simulink model "bpsk_revised"  (R2024a)
settings: Solver=FixedStepAuto  StartTime=0.0  StopTime=100  FixedStep=1e-3  RelTol=1e-3
libraries: dspfdesign x2, simulink x1, commutil2 x1, dspsigops x1, commdigbbndpm3 x1, dspsrcs4 x1
settings Model: DataTypeOverride=Off  Creator=Alang  LastModifiedBy=andy1
settings SolverCC: AlgebraicLoopSolver=TrustRegion  AutoInsertRateTranBlk=on
settings DataIOCC: SaveOutput=off  SaveTime=off
settings OptimizationCC: BlockReduction=off  ConditionallyExecuteInputs=off  DefaultParameterBehavior=Inlined  LifeSpan=inf
settings DebuggingCC: AlgebraicLoopMsg=error  SingleTaskRateTransMsg=error  UnconnectedInputMsg=warning  UnconnectedOutputMsg=warning  UnconnectedLineMsg=warning  AllowSymbolicDim=off  StrictBusMsg=ErrorOnBusTreatedAsVector  SFUnexpectedBacktrackingDiag=warning  SFNoUnconditionalDefaultTransitionDiag=warning  SFExecutionAtInitializationDiag=none  ArithmeticOperatorsInVariantConditions=warning
settings HardwareCC: ProdBitPerPointer=32  ProdBitPerSizeT=32  ProdBitPerPtrDiffT=32  ProdLargestAtomicFloat=None  ProdIntDivRoundTo=Undefined  ProdEndianess=Unspecified  ProdWordSize=32  ProdHWDeviceType=ASIC/FPGA->ASIC/FPGA  ProdEqTarget=off
settings ModelReferenceCC: EnableRefExpFcnMdlSchedulingChecks=on
settings SFSimCC: SimUseLocalCustomCode=off  CustomCodeUndefinedFunction=UseInterfaceOnly
settings RTWCC: RTWUseLocalCustomCode=off  GPUComputeCapability=3.5  DLArmComputeVersion=19.05
settings CodeAppCC: StateflowObjectComments=on
settings GRTTargetCC: TargetLangStandard=C89/C90 (ANSI)
settings ConfigComp: CovScope=ReferencedModels  CovMetricSettings=dw  CovSaveCumulativeToWorkspaceVar=on  CovSaveSingleToWorkspaceVar=on  CovExternalEMLEnable=off  CovSFcnEnable=off

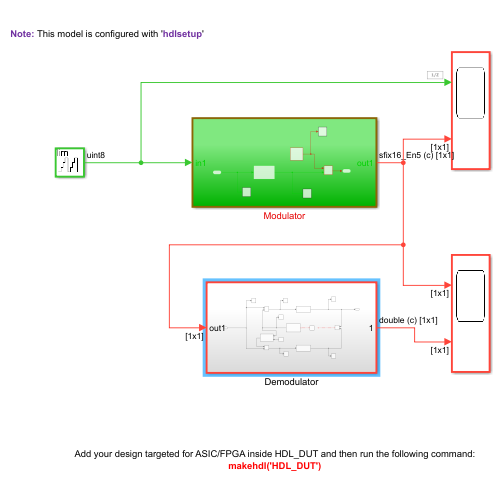
[thumbnail: Simulink's stored preview of the top-level diagram]
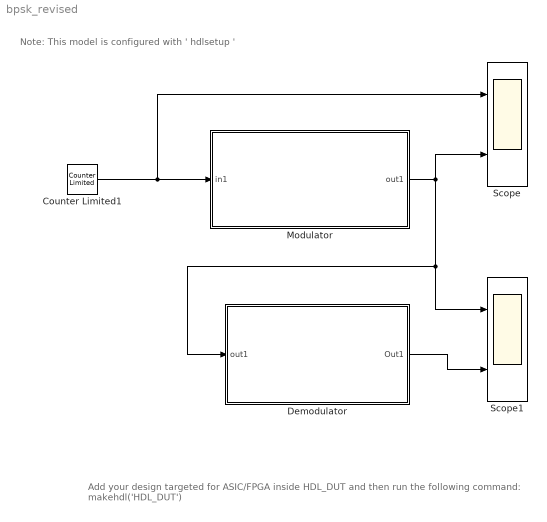
== system bpsk_revised ==
  note: Note: This model is configured with ' hdlsetup '
  note: Add your design targeted for ASIC/FPGA inside HDL_DUT and then run the following command:
      | makehdl('HDL_DUT')
  Counter Limited1 : simulink/Sources/Counter Limited  uplimit=1  tsamp=1
  Demodulator : Subsystem
  Modulator : Subsystem
  Scope : Scope  NumInputPorts=2
  Scope1 : Scope  NumInputPorts=2
  wires:
  Modulator/1(out1) -> Scope1/1, Demodulator/1(out1), Scope/2
  Counter Limited1/1 -> Modulator/1(in1), Scope/1
  Demodulator/1(Out1) -> Scope1/2

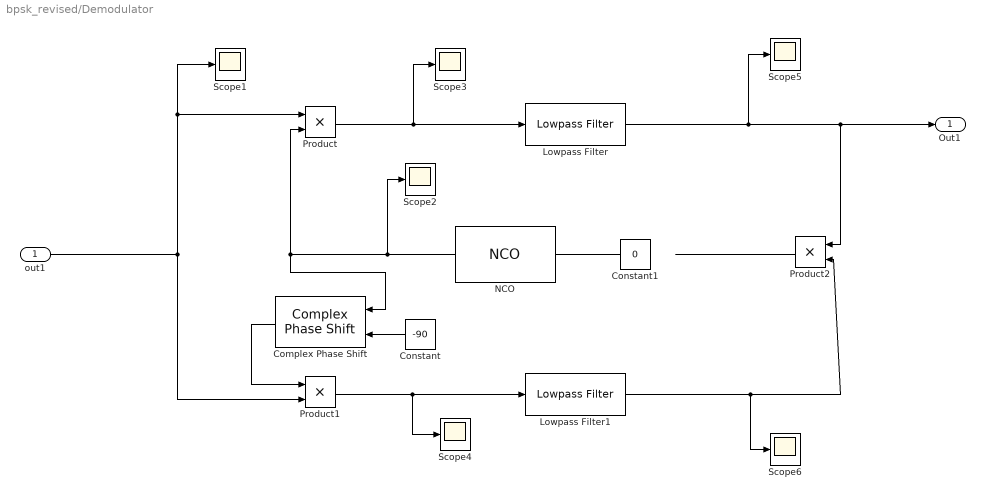
== system bpsk_revised/Demodulator ==
  out1 : Inport
  Complex Phase Shift : commutil2/Complex Phase Shift
  Constant : Constant  Value=-90  OutDataTypeStr=double
  Constant1 : Constant  Value=0  OutDataTypeStr=int8
  Lowpass Filter : dspfdesign/Lowpass Filter  FilterType=FIR  DesignForMinimumOrder=on  FilterOrder=50  PassbandFrequency=8e3  StopbandFrequency=12e3  PassbandRipple=0.1  StopbandAttenuation=80  SampleRateMode=Specify on dialog  SampleRate=44100  SimulateUsing=Interpreted execution  roundingMode=Floor  coeffsDataTypeStr=fixdt(1,16)
  Lowpass Filter1 : dspfdesign/Lowpass Filter  FilterType=FIR  DesignForMinimumOrder=on  FilterOrder=50  PassbandFrequency=8e3  StopbandFrequency=12e3  PassbandRipple=0.1  StopbandAttenuation=80  SampleRateMode=Specify on dialog  SampleRate=44100  SimulateUsing=Interpreted execution  roundingMode=Floor  coeffsDataTypeStr=fixdt(1,16)
  NCO : dspsigops/NCO  AccIncSrc=Specify via dialog  AccInc=65  PhaseOffsetSrc=Specify via dialog  PhaseOffset=0  AccumWL=16  HasDither=off  DitherWL=4  PNgeneratorLength=19  HasPhaseQuantizer=on  TableDepth=12  HasOutputPhaseError=off  Formula=Sine  DataType=double  OutputWL=16  OutputFL=14  CompMethod=Table lookup (no interpolation)  SampleTime=0.001  SamplesPerFrame=1  OutputFrames=off
      settings: LibrarySourceBlock=dspsrcs4/NCO
  Product : Product
  Product1 : Product
  Product2 : Product
  Scope{1..6} (6 alike) : Scope
  Out1 : Outport
  wires:
  out1/1 -> Product/1, Scope1/1, Product1/2
  Lowpass Filter/1 -> Scope5/1, Product2/1, Out1/1
  Lowpass Filter1/1 -> Scope6/1, Product2/2
  Complex Phase Shift/1 -> Product1/1
  NCO/1 -> Scope2/1, Product/2, Complex Phase Shift/1
  Constant/1 -> Complex Phase Shift/2
  Product2/1 -> ?
  Constant1/1 -> ?
  Product1/1 -> Scope4/1, Lowpass Filter1/1
  Product/1 -> Scope3/1, Lowpass Filter/1

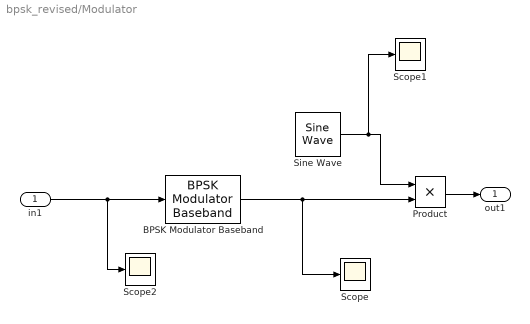
== system bpsk_revised/Modulator ==
  in1 : Inport
  BPSK Modulator Baseband : commdigbbndpm3/BPSK Modulator Baseband  Ph=0  outDtype=Fixed-point  outWordLen=16  outUDDataType=sfix(16)  outFracLenMode=Best precision  outFracLen=15  outDataTypeStr=fixdt(1,16)  outLastDataTypeStr=fixdt(1,16)
  Product : Product  OutMin=[0]  OutMax=[1000]  OutDataTypeStr=fixdt(1,16)
  Scope : Scope
  Scope1 : Scope
  Scope2 : Scope
  Sine Wave : dspsrcs4/Sine Wave  Amplitude=1  Frequency=10  Phase=pi/2  SampleMode=Discrete  OutComplex=Real  CompMethod=Table lookup  TableSize=Speed  SampleTime=1/1000  SamplesPerFrame=1  ResetState=Restart at time zero  OutputFrames=off  dataType=Fixed-point  wordLen=16  udDataType=sfix(16)  fracBitsMode=Best precision  numFracBits=14  OutDataTypeStr=fixdt(1,16)  LastOutDataTypeStr=fixdt(1,16)
  out1 : Outport  VectorParamsAs1DForOutWhenUnconnected=off
  wires:
  in1/1 -> Scope2/1, BPSK Modulator Baseband/1
  BPSK Modulator Baseband/1 -> Scope/1, Product/2
  Sine Wave/1 -> Scope1/1, Product/1
  Product/1 -> out1/1
